simulink model "q2_D"  (R2016b)
settings: Solver=VariableStepAuto  StartTime=0.0  StopTime=100  RelTol=1e-3
libraries: simulink_extras x4
settings Model: Creator=dell  LastModifiedBy=dell
settings OptimizationCC: BooleanDataType=off

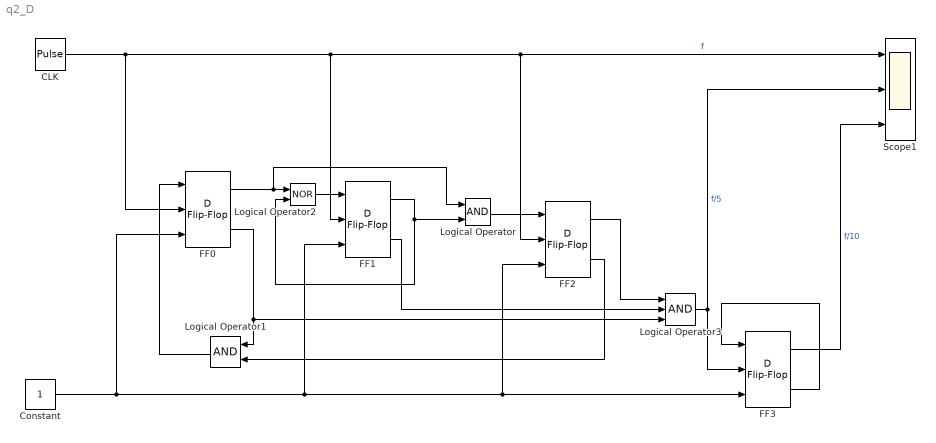
== system q2_D ==
  CLK : DiscretePulseGenerator  Period=6  PulseWidth=3
  Constant : Constant  OutDataTypeStr=boolean
  FF{0..3} (4 alike) : simulink_extras/Flip Flops/D Flip-Flop
  Logical Operator : Logic  AllPortsSameDT=off  OutDataTypeStr=boolean
  Logical Operator1 : Logic  AllPortsSameDT=off  OutDataTypeStr=boolean
  Logical Operator2 : Logic  Operator=NOR  AllPortsSameDT=off  OutDataTypeStr=boolean
  Logical Operator3 : Logic  Inputs=3  AllPortsSameDT=off  OutDataTypeStr=boolean
  Scope1 : Scope  NumInputPorts=3
  wires:
  Logical Operator1/1 -> FF0/1
  Logical Operator/1 -> FF2/1
  FF1/1 -> Logical Operator2/2, Logical Operator/2
  FF0/1 -> Logical Operator/1, Logical Operator2/1
  Logical Operator2/1 -> FF1/1
  Constant/1 -> FF0/3, FF2/3, FF3/3, FF1/3
  CLK/1 -> FF1/2, Scope1/1, FF2/2, FF0/2  "f"
  Logical Operator3/1 -> Scope1/2, FF3/2  "f/5"
  FF2/1 -> Logical Operator3/1
  FF1/2 -> Logical Operator3/2
  FF0/2 -> Logical Operator3/3, Logical Operator1/1
  FF3/1 -> Scope1/3  "f/10"
  FF3/2 -> FF3/1
  FF2/2 -> Logical Operator1/2
